simulink model "LQG_AWBT_Algorithm7"  (R2015a)
settings: Solver=ode5  StartTime=0.0  StopTime=80  FixedStep=5e-5  RelTol=1e-3
values from neighbouring files (symbols this model uses):
  Ac = [-58.0981835397 -4179.57477778 -14.3009592549 -19.6551859971 -26.1377959927 51.7079073443 78.2309892718 -133.106022928 -125.54564289 -182.0885271 37.0670033238 40.9567129567 ... (144 elements, 12x12)]    [controller.mat]    (also in main_matlab_Anderson.m = rlqg.A; main_matlab_LMI_Algorithm2.m = rlqg.A; main_matlab_LMI_Algorithm4.m = rlqg.A; main_matlab_LMI_Algorithm6.m = rlqg.A)
  Ap = A    [main_matlab_Anderson.m]    (also in main_matlab_LMI_Algorithm2.m; main_matlab_LMI_Algorithm4.m; main_matlab_LMI_Algorithm6.m; main_matlab_LMI_Algorithm7.m)
  Bc = [0.70645219319 -0.459324928491 1.97272580341 3.24573294172 13.9295718254 5.65537256369 -43.2723544643 48.5060616978 79.1032122304 114.834038365 0.0916332028948 -11.1940741965]    [controller.mat]    (also in main_matlab_Anderson.m = rlqg.B; main_matlab_LMI_Algorithm2.m = rlqg.B; main_matlab_LMI_Algorithm4.m = rlqg.B; main_matlab_LMI_Algorithm6.m = rlqg.B)
  Bpu = B    [main_matlab_Anderson.m]    (also in main_matlab_LMI_Algorithm2.m; main_matlab_LMI_Algorithm4.m; main_matlab_LMI_Algorithm6.m; main_matlab_LMI_Algorithm7.m)
  Cc = [64.5329237696 -12.8289022427 -137.386503701 73.2919038483 43.4280804178 151.107833676 54.9118478641 123.622857411 -29.577337272 16.1677085133 -56.2730534034 204.335066283 ... (24 elements, 2x12)]    [controller.mat]    (also in main_matlab_Anderson.m = rlqg.C; main_matlab_LMI_Algorithm2.m = rlqg.C; main_matlab_LMI_Algorithm4.m = rlqg.C; main_matlab_LMI_Algorithm6.m = rlqg.C)
  Dc = [0 0]    [controller.mat]    (also in main_matlab_Anderson.m = rlqg.D; main_matlab_LMI_Algorithm2.m = rlqg.D; main_matlab_LMI_Algorithm4.m = rlqg.D; main_matlab_LMI_Algorithm6.m = rlqg.D)
  K = X1*inv(Q)    [main_matlab_LMI_Algorithm7.m]
  L = X2*inv(U)    [main_matlab_LMI_Algorithm7.m]
  ub = 100    [main_matlab_LMI_Algorithm7.m]
undefined symbols (not defined in the file or in its folder): Af, Bf, Cf, Hf
libraries: simulink x1, cstblocks x1
settings Model: Creator=p4wp4w  LastModifiedBy=Ablah

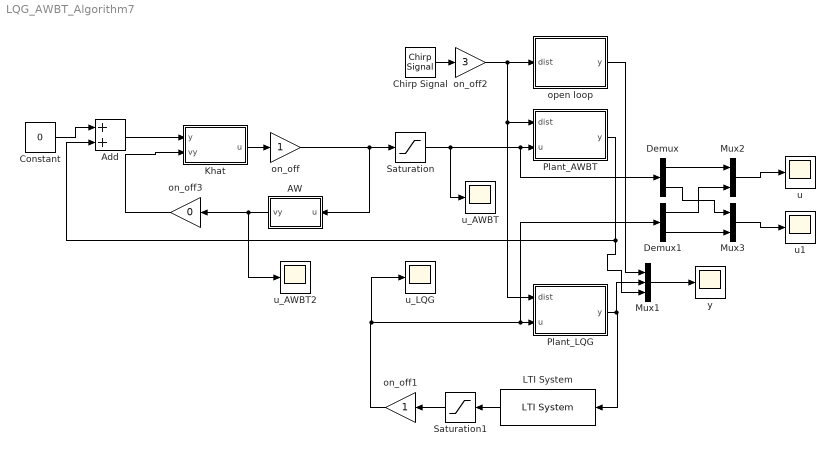
== system LQG_AWBT_Algorithm7 ==
  AW : Subsystem
  Add : Sum
  Chirp Signal : simulink/Sources/Chirp Signal  f1=0.1  T=80  f2=800
  Constant : Constant  Value=0
  Demux : Demux  Outputs=2
  Demux1 : Demux  Outputs=2
  Khat : Subsystem
  LTI System : cstblocks/LTI System  sys=rlqg  IC=[]
  Mux1 : Mux  Inputs=3
  Mux2 : Mux  Inputs=2
  Mux3 : Mux  Inputs=2
  Plant_AWBT : Subsystem
  Plant_LQG : Subsystem
  Saturation : Saturate  UpperLimit=ub  LowerLimit=-ub
  Saturation1 : Saturate  UpperLimit=ub  LowerLimit=-ub
  on_off : Gain
  on_off1 : Gain
  on_off2 : Gain  Gain=3
  on_off3 : Gain  Gain=0
  open loop : Subsystem
  u : Scope
      settings: ShowLegends=on  YMin=-0.8  YMax=0.7  SaveName=ScopeData3
  u1 : Scope
      settings: ShowLegends=on  YMin=-0.8  YMax=0.7  SaveName=ScopeData5
  u_AWBT : Scope
      settings: YMin=-75  YMax=100
  u_AWBT2 : Scope
      settings: YMin=-150  YMax=150  SaveName=ScopeData4
  u_LQG : Scope
      settings: SaveName=ScopeData2
  y : Scope
      settings: ShowLegends=on  YMin=-15  YMax=15
  wires:
  Khat/1("u ") -> on_off/1
  Saturation/1 -> u_AWBT/1, Demux/1, Plant_AWBT/2(u)
  on_off/1 -> AW/1(u), Saturation/1
  Chirp Signal/1 -> on_off2/1
  LTI System/1 -> Saturation1/1
  Saturation1/1 -> on_off1/1
  Mux1/1 -> y/1
  open loop/1(y) -> Mux1/1
  on_off1/1 -> u_LQG/1, Demux1/1, Plant_LQG/2(u)
  AW/1(vy) -> u_AWBT2/1, on_off3/1
  on_off2/1 -> open loop/1(dist), Plant_LQG/1(dist), Plant_AWBT/1(dist)
  Plant_LQG/1(y) -> Mux1/2, LTI System/1
  Plant_AWBT/1(y) -> Add/2, Mux1/3
  Demux/1 -> Mux2/1
  Demux1/1 -> Mux2/2
  Demux/2 -> Mux3/1
  Demux1/2 -> Mux3/2
  Mux3/1 -> u1/1
  Mux2/1 -> u/1
  Add/1 -> Khat/1(y)
  Constant/1 -> Add/1
  on_off3/1 -> Khat/2("vy ")

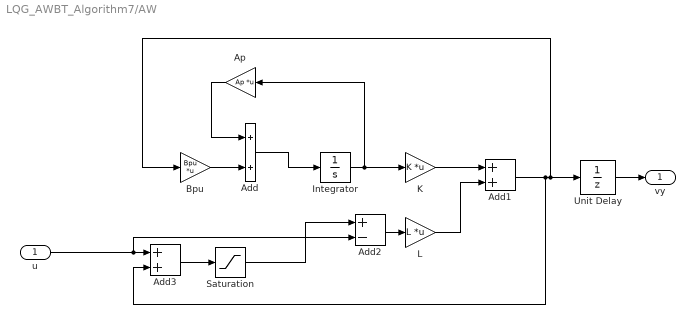
== system LQG_AWBT_Algorithm7/AW ==
  u : Inport
  Add : Sum
  Add1 : Sum
  Add2 : Sum  Inputs=+-
  Add3 : Sum
  Ap : Gain  Gain=Ap  Multiplication=Matrix(K*u)
  Bpu : Gain  Gain=Bpu  Multiplication=Matrix(K*u)
  Integrator : Integrator
  K : Gain  Gain=K  Multiplication=Matrix(K*u)
  L : Gain  Gain=L  Multiplication=Matrix(K*u)
  Saturation : Saturate  UpperLimit=ub  LowerLimit=-ub
  Unit Delay : UnitDelay  SampleTime=-1
  vy : Outport
  wires:
  Add/1 -> Integrator/1
  Ap/1 -> Add/1
  Integrator/1 -> K/1, Ap/1
  K/1 -> Add1/1
  L/1 -> Add1/2
  Add2/1 -> L/1
  u/1 -> Add2/2, Add3/1
  Add3/1 -> Saturation/1
  Saturation/1 -> Add2/1
  Bpu/1 -> Add/2
  Add1/1 -> Add3/2, Bpu/1, Unit Delay/1
  Unit Delay/1 -> vy/1

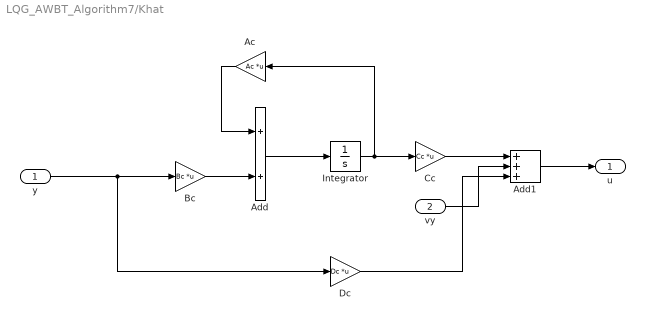
== system LQG_AWBT_Algorithm7/Khat ==
  y : Inport
  "vy " : Inport  Port=2
  Ac : Gain  Gain=Ac  Multiplication=Matrix(K*u)
  Add : Sum
  Add1 : Sum  Inputs=+++
  Bc : Gain  Gain=Bc  Multiplication=Matrix(K*u)
  Cc : Gain  Gain=Cc  Multiplication=Matrix(K*u)
  Dc : Gain  Gain=Dc  Multiplication=Matrix(K*u)
  Integrator : Integrator
  "u " : Outport
  wires:
  Add/1 -> Integrator/1
  Bc/1 -> Add/2
  Ac/1 -> Add/1
  y/1 -> Dc/1, Bc/1
  Integrator/1 -> Ac/1, Cc/1
  Cc/1 -> Add1/1
  "vy "/1 -> Add1/2
  Dc/1 -> Add1/3
  Add1/1 -> "u "/1

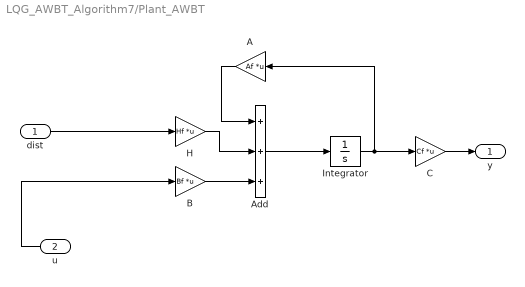
== system LQG_AWBT_Algorithm7/Plant_AWBT ==
  dist : Inport
  u : Inport  Port=2
  A : Gain  Gain=Af  Multiplication=Matrix(K*u)
  Add : Sum  Inputs=+++
  B : Gain  Gain=Bf  Multiplication=Matrix(K*u)
  C : Gain  Gain=Cf  Multiplication=Matrix(K*u)
  H : Gain  Gain=Hf  Multiplication=Matrix(K*u)
  Integrator : Integrator
  y : Outport
  wires:
  Add/1 -> Integrator/1
  H/1 -> Add/2
  A/1 -> Add/1
  dist/1 -> H/1
  C/1 -> y/1
  B/1 -> Add/3
  Integrator/1 -> C/1, A/1
  u/1 -> B/1

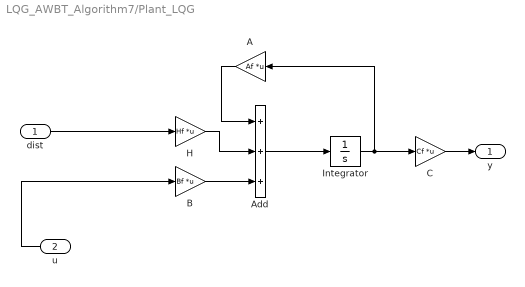
== system LQG_AWBT_Algorithm7/Plant_LQG ==
  dist : Inport
  u : Inport  Port=2
  A : Gain  Gain=Af  Multiplication=Matrix(K*u)
  Add : Sum  Inputs=+++
  B : Gain  Gain=Bf  Multiplication=Matrix(K*u)
  C : Gain  Gain=Cf  Multiplication=Matrix(K*u)
  H : Gain  Gain=Hf  Multiplication=Matrix(K*u)
  Integrator : Integrator
  y : Outport
  wires:
  u/1 -> B/1
  Integrator/1 -> A/1, C/1
  B/1 -> Add/3
  C/1 -> y/1
  dist/1 -> H/1
  A/1 -> Add/1
  H/1 -> Add/2
  Add/1 -> Integrator/1

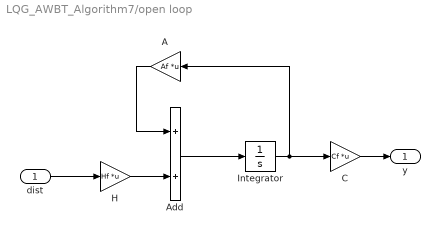
== system LQG_AWBT_Algorithm7/open loop ==
  dist : Inport
  A : Gain  Gain=Af  Multiplication=Matrix(K*u)
  Add : Sum
  C : Gain  Gain=Cf  Multiplication=Matrix(K*u)
  H : Gain  Gain=Hf  Multiplication=Matrix(K*u)
  Integrator : Integrator
  y : Outport
  wires:
  Integrator/1 -> A/1, C/1
  C/1 -> y/1
  dist/1 -> H/1
  A/1 -> Add/1
  H/1 -> Add/2
  Add/1 -> Integrator/1
